simulink library "create_THB"  (Simulink 8.2)
settings: Solver=ode45  StartTime=0.0  StopTime=10.0  RelTol=1e-3
libraries: carnot x1
settings Model: Creator=lena.frank  LastModifiedBy=awohlfei

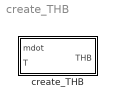
== system create_THB ==
  create_THB : Subsystem  InitFcn=load('THB.mat');  mask(create THB){p=1e5, fluid=Water, mix=0, dia=0.02, mID=No Pressure Drop}
      mask prompts: p "pressure [Pa]"; mix "fluid mixture [0..1]"; dia "diameter [m]"; mID "Caclulation mode"
      mask help: Block to create a THB with the variable input T and mdot. The other value can be set as constants in the mask.
      mask init:
      | mix = min(1, max(0, mix));
      | dia = max(dia, 0.001);
      | ID = (mID-1)*10000+1;
      mask Help: web(fullfile(path_carnot('help'),'createTHB.html'),'-helpbrowser')
      mask TypeOptions fluid: Water | Air | Cotton Oil | Silicone Oil | Water-Glycol Mix | Tyfocor LS | Water (Constant 20°C) | Air (dry+ constant 20°C)
      mask TypeOptions mID: No Pressure Drop | Pressure Drop from Massflow | Full Pressure Drop with Static Height

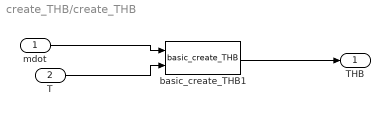
== system create_THB/create_THB ==
  mdot : Inport
  T : Inport  Port=2
  basic_create_THB1 : carnot/Basic/Hydraulics/basic_create_THB  p=p  fluid=fluid  mix=mix  dia=dia  hgt=0  mID=mID
  THB : Outport
  wires:
  T/1 -> basic_create_THB1/2
  basic_create_THB1/1 -> THB/1
  mdot/1 -> basic_create_THB1/1
